simulink model "purePursuitCurveHighVel"  (R2021b)
settings: Solver=ode3  StartTime=0.0  StopTime=Ts2  FixedStep=0.01  RelTol=1e-3
PreLoadFcn:
  | setUpPurePursuitCurveHighVel
model workspace (MAT data in the model file):
  firstWarning = 0
  originalScenarioChecksum = 'F73A6DA3C723D3CA73A6F931B7A52A9C'
values from neighbouring files (symbols this model uses):
  L = 1.524    [matlab.mat]    (also in matlab2.mat)
  ld = 2    [matlab.mat]    (also in matlab2.mat)
  lr = 0.838    [matlab.mat]    (also in matlab2.mat)
  m = 300    [matlab.mat]    (also in matlab2.mat)
  Rw = 0.265    [matlab.mat]    (also in matlab2.mat)
  s = [73 1]    [matlab.mat]    (also in matlab2.mat)
  tr = 0.549    [matlab.mat]    (also in matlab2.mat)
  v_des = 20    [matlab.mat]    (also in matlab2.mat)
  X_o = 0    [matlab.mat]    (also in matlab2.mat)
  xRef2 = [0 1 2 3 4 5 6 7 8 9 10 11 ... (225 elements, 225x1)]    [matlab.mat]    (also in matlab2.mat)
  Y_o = 0    [matlab.mat]    (also in matlab2.mat)
  yRef2 = [0 0 0 0 0 0 0 0 0 0 0 0.5 ... (225 elements, 225x1)]    [matlab.mat]    (also in matlab2.mat)
undefined symbols (not defined in the file or in its folder): MMax, psi_o
libraries: autolibutils x4, autolibshared x3, vehdynlibviscommon x1, simulink_extras x1, vehdynlibsteering x1, robotalgslib x1, simulink x1
(part 3 of 3)

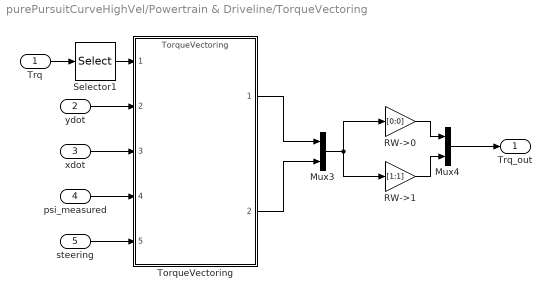
== system purePursuitCurveHighVel/Powertrain & Driveline/TorqueVectoring ==
  Trq : Inport
  ydot : Inport  Port=2
  xdot : Inport  Port=3
  psi_measured : Inport  Port=4
  steering : Inport  Port=5
  Mux3 : Mux  Inputs=2
  Mux4 : Mux  Inputs=2
  RW->0 : Gain  Gain=[0;0]
  RW->1 : Gain  Gain=[1;1]
  Selector1 : Selector  InputPortWidth=4  IndexOptions=Index vector (dialog)  Indices=[3]  OutputSizes=1
  TorqueVectoring : ModelReference  ModelNameDialog=TorqueVectoring  SimulationMode=Normal  ModelReferenceVersion=4.11
  Trq_out : Outport  OutDataTypeStr=double  PortDimensions=4  SampleTime=0
  wires:
  psi_measured/1 -> TorqueVectoring/4
  Trq/1 -> Selector1/1
  xdot/1 -> TorqueVectoring/3
  ydot/1 -> TorqueVectoring/2
  steering/1 -> TorqueVectoring/5
  TorqueVectoring/1 -> Mux3/1
  RW->0/1 -> Mux4/1
  TorqueVectoring/2 -> Mux3/2
  Mux4/1 -> Trq_out/1
  RW->1/1 -> Mux4/2
  Mux3/1 -> RW->1/1, RW->0/1
  Selector1/1 -> TorqueVectoring/1

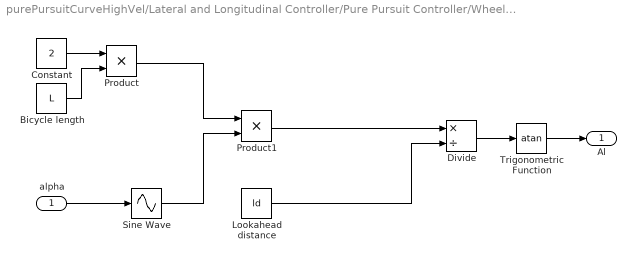
== system purePursuitCurveHighVel/Lateral and Longitudinal Controller/Pure Pursuit Controller/Wheel Steering Angle Formulation ==
  alpha : Inport
  Bicycle length : Constant  Value=L
  Constant : Constant  Value=2
  Divide : Product  Inputs=*/
  Lookahead distance : Constant  Value=ld
  Product : Product
  Product1 : Product
  Sine Wave : Sin  TimeSource=Use external signal  SampleTime=0
  Trigonometric Function : Trigonometry  Operator=atan
  Al : Outport
  wires:
  Sine Wave/1 -> Product1/2
  Bicycle length/1 -> Product/2
  Constant/1 -> Product/1
  Product1/1 -> Divide/1
  Product/1 -> Product1/1
  Divide/1 -> Trigonometric Function/1
  Trigonometric Function/1 -> Al/1
  alpha/1 -> Sine Wave/1
  Lookahead distance/1 -> Divide/2

== system purePursuitCurveHighVel/Powertrain & Driveline/Driveline/RWD ==
  TPowertrain : Inport
  RWD : Gain  Gain=[0;0;1;1]
  TAxles : Outport  VectorParamsAs1DForOutWhenUnconnected=off
  wires:
  TPowertrain/1 -> RWD/1
  RWD/1 -> TAxles/1

== matlab function purePursuitCurveHighVel/Powertrain & Driveline/TrqDistribution ==
  data: vLa input; vRa input; vL output; vR output; vx input; c input
function [vL,vR] = fcn(vLa,vRa,vx, c)
%#codegen

if vLa <= vx 
    vL = vLa* (1+ c);
else
    vL = vLa* (1- c);
end

if vRa <= vx
    vR = vRa* (1+ c);
else
    vR = vRa* (1- c);
end
